simulink model "two_virtual_wheel_subsystems"  (Simulink 7.8)
settings: Solver=FixedStepDiscrete  SolverMode=MultiTasking  StartTime=0.0  StopTime=tfinal  RelTol=1e-3
InitFcn:
  | two_virtual_wheel_params
undefined symbols (not defined in the file): b1, b2, DiscIntNeverNeededParam, Jw1, Jw2, k1, k2, step_time, Theta_z_0
libraries: simulink x2
settings Model: Creator=Embed_Sys_course  LastModifiedBy=Embed_Sys_course  ExtModeTrigMode=oneshot  ExtModeArmWhenConnect=off
settings DataIOCC: LimitDataPoints=off  SignalLoggingName=sigsOut
settings OptimizationCC: BooleanDataType=off  InitFltsAndDblsToZero=on
settings DebuggingCC: SaveWithParameterizedLinksMsg=none  SignalResolutionControl=TryResolveAllWithWarning  SolverPrmCheckMsg=none  MultiTaskDSMMsg=warning  MultiTaskCondExecSysMsg=none  FcnCallInpInsideContextMsg=Use local settings  StrictBusMsg=None
settings HardwareCC: TargetIntDivRoundTo=Zero  TargetEndianess=LittleEndian  TargetHWDeviceType=MATLAB Host  ProdEqTarget=off
settings RTWCC: IncludeERTFirstTime=on
settings GRTTargetCC: TargetFcnLib=ansi_tfl_tmw.mat

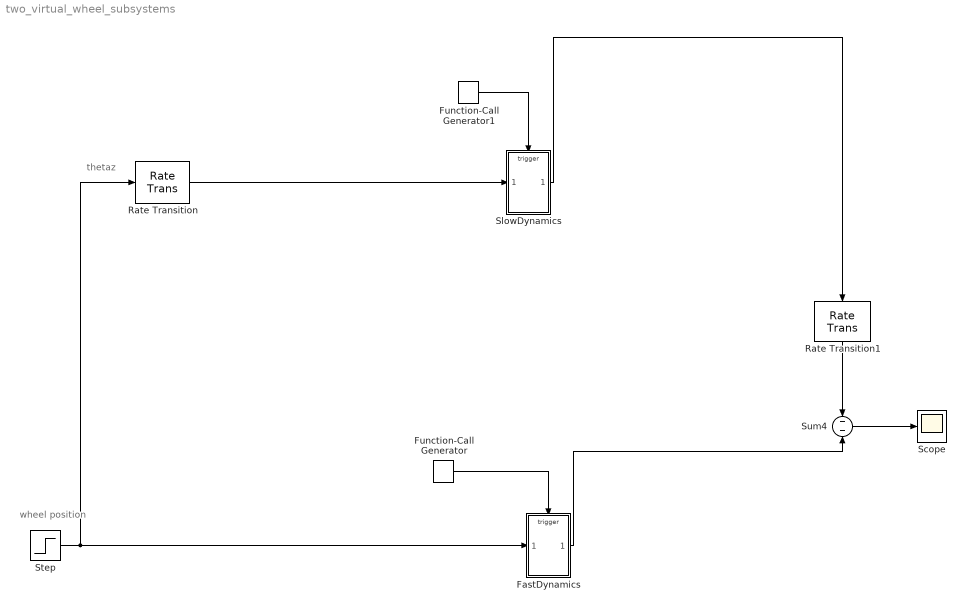
== system two_virtual_wheel_subsystems ==
  note: wheel position
  note: thetaz
  FastDynamics : Subsystem
  Function-Call Generator : simulink/Ports & Subsystems/Function-Call Generator  sample_time=0.002  numberOfIterations=1
  Function-Call Generator1 : simulink/Ports & Subsystems/Function-Call Generator  sample_time=0.02  numberOfIterations=1
  Rate Transition : RateTransition
  Rate Transition1 : RateTransition
  Scope : Scope
  SlowDynamics : Subsystem
  Step : Step  Time=step_time  After=Theta_z_0
  Sum4 : Sum  Inputs=-|-  SaturateOnIntegerOverflow=on  InputSameDT=on  OutDataTypeStr=Inherit: Same as first input
  wires:
  Step/1 -> Rate Transition/1, FastDynamics/1(In1)
  Sum4/1 -> Scope/1
  Rate Transition1/1 -> Sum4/1
  Rate Transition/1 -> SlowDynamics/1(thetaz)
  SlowDynamics/1(torque1) -> Rate Transition1/1
  FastDynamics/1(torque2) -> Sum4/2
  Function-Call Generator1/1 -> SlowDynamics/Trigger
  Function-Call Generator/1 -> FastDynamics/Trigger

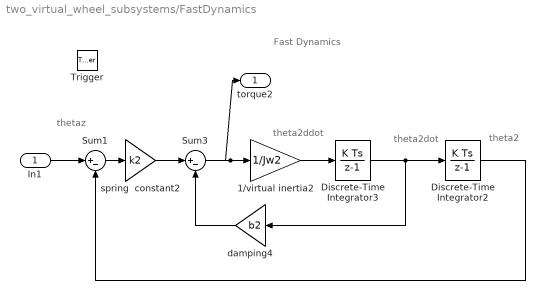
== system two_virtual_wheel_subsystems/FastDynamics ==
  note: Fast Dynamics
  note: thetaz
  note: theta2ddot
  note: theta2dot
  note: theta2
  In1 : Inport
  Trigger : TriggerPort  TriggerType=function-call  PortDimensions=1
  1/virtual inertia2 : Gain  Gain=1/Jw2  SaturateOnIntegerOverflow=on  OutDataTypeStr=Inherit: Same as input  ParamDataTypeStr=Inherit: Same as input
  Discrete-Time Integrator2 : DiscreteIntegrator  SampleTime=-1  ICPrevOutput=DiscIntNeverNeededParam  ICPrevScaledInput=DiscIntNeverNeededParam
  Discrete-Time Integrator3 : DiscreteIntegrator  SampleTime=-1  ICPrevOutput=DiscIntNeverNeededParam  ICPrevScaledInput=DiscIntNeverNeededParam
  Sum1 : Sum  Inputs=|+-  SaturateOnIntegerOverflow=on  InputSameDT=on  OutDataTypeStr=Inherit: Same as first input
  Sum3 : Sum  Inputs=|+-  SaturateOnIntegerOverflow=on  InputSameDT=on  OutDataTypeStr=Inherit: Same as first input
  damping4 : Gain  Gain=b2  SaturateOnIntegerOverflow=on  OutDataTypeStr=Inherit: Same as input  ParamDataTypeStr=Inherit: Same as input
  spring  constant2 : Gain  Gain=k2  SaturateOnIntegerOverflow=on  OutDataTypeStr=Inherit: Same as input  ParamDataTypeStr=Inherit: Same as input
  torque2 : Outport
  wires:
  spring  constant2/1 -> Sum3/1
  damping4/1 -> Sum3/2
  Sum3/1 -> torque2/1, 1/virtual inertia2/1
  Discrete-Time Integrator3/1 -> Discrete-Time Integrator2/1, damping4/1
  1/virtual inertia2/1 -> Discrete-Time Integrator3/1
  Sum1/1 -> spring  constant2/1
  Discrete-Time Integrator2/1 -> Sum1/2
  In1/1 -> Sum1/1

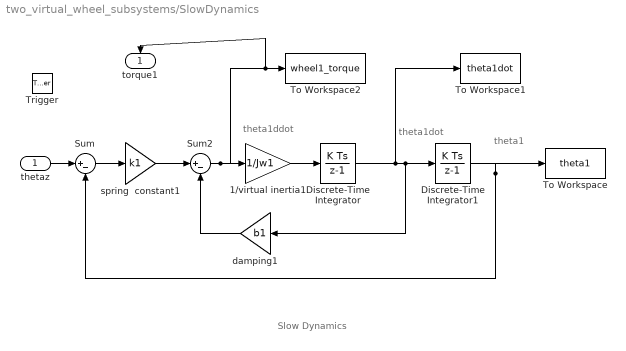
== system two_virtual_wheel_subsystems/SlowDynamics ==
  note: Slow Dynamics
  note: theta1ddot
  note: theta1dot
  note: theta1
  thetaz : Inport
  Trigger : TriggerPort  TriggerType=function-call  PortDimensions=1
  1/virtual inertia1 : Gain  Gain=1/Jw1  SaturateOnIntegerOverflow=on  OutDataTypeStr=Inherit: Same as input  ParamDataTypeStr=Inherit: Same as input
  Discrete-Time Integrator : DiscreteIntegrator  SampleTime=-1  ICPrevOutput=DiscIntNeverNeededParam  ICPrevScaledInput=DiscIntNeverNeededParam
  Discrete-Time Integrator1 : DiscreteIntegrator  SampleTime=-1  ICPrevOutput=DiscIntNeverNeededParam  ICPrevScaledInput=DiscIntNeverNeededParam
  Sum : Sum  Inputs=|+-  SaturateOnIntegerOverflow=on  InputSameDT=on  OutDataTypeStr=Inherit: Same as first input
  Sum2 : Sum  Inputs=|+-  SaturateOnIntegerOverflow=on  InputSameDT=on  OutDataTypeStr=Inherit: Same as first input
  To Workspace : ToWorkspace  VariableName=theta1  SampleTime=-1  SaveFormat=Structure With Time
  To Workspace1 : ToWorkspace  VariableName=theta1dot  SampleTime=-1  SaveFormat=Structure With Time
  To Workspace2 : ToWorkspace  VariableName=wheel1_torque  SampleTime=-1  SaveFormat=Structure With Time
  damping1 : Gain  Gain=b1  SaturateOnIntegerOverflow=on  OutDataTypeStr=Inherit: Same as input  ParamDataTypeStr=Inherit: Same as input
  spring  constant1 : Gain  Gain=k1  SaturateOnIntegerOverflow=on  OutDataTypeStr=Inherit: Same as input  ParamDataTypeStr=Inherit: Same as input
  torque1 : Outport
  wires:
  damping1/1 -> Sum2/2
  Sum2/1 -> 1/virtual inertia1/1, To Workspace2/1, torque1/1
  spring  constant1/1 -> Sum2/1
  Discrete-Time Integrator/1 -> Discrete-Time Integrator1/1, damping1/1, To Workspace1/1
  1/virtual inertia1/1 -> Discrete-Time Integrator/1
  Sum/1 -> spring  constant1/1
  Discrete-Time Integrator1/1 -> Sum/2, To Workspace/1
  thetaz/1 -> Sum/1
